simulink model "scheme1"  (R2014a)
settings: Solver=ode45  StartTime=0.0  StopTime=100  MaxStep=0.001  MinStep=0.0001  RelTol=1e-3
settings Model: Creator=User  LastModifiedBy=trigg

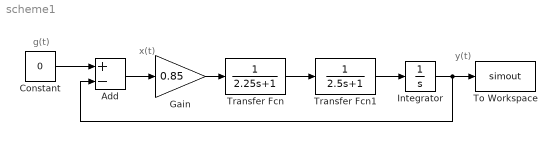
== system scheme1 ==
  note: y(t)
  note: x(t)
  note: g(t)
  Add : Sum  Inputs=+-
  Constant : Constant  Value=0
  Gain : Gain  Gain=0.85
  Integrator : Integrator  InitialCondition=1
  To Workspace : ToWorkspace  VariableName=simout  SaveFormat=Timeseries  SampleTime=-1
  Transfer Fcn : TransferFcn  Denominator=[2.25 1]
  Transfer Fcn1 : TransferFcn  Denominator=[2.5 1]
  wires:
  Transfer Fcn1/1 -> Integrator/1
  Transfer Fcn/1 -> Transfer Fcn1/1
  Gain/1 -> Transfer Fcn/1
  Add/1 -> Gain/1
  Integrator/1 -> To Workspace/1, Add/2
  Constant/1 -> Add/1
